simulink model "Controllo_Dinamica_Inversa_Spazio_Operativo"  (R2023a)
settings: Solver=VariableStepAuto  StartTime=0.0  StopTime=113  RelTol=1e-3
values from neighbouring files (symbols this model uses):
  a1 = 0.5    [Progetto_FoR.m]
  d0 = 1    [Progetto_FoR.m]
  KD4 = diag(kd4)    [Progetto_FoR.m]
  KI = diag(ki)    [Progetto_FoR.m]
  KP4 = diag(kp4)    [Progetto_FoR.m]
  pi0 = [ml1 Il1 Im1 Fm1 ml2 Il2 Im2 Fm2 ml3 Im3 Fm3 Il4 Im4 Fm4]    [Progetto_FoR.m]
  q0 = [0 pi/2 0 pi/2]    [Progetto_FoR.m]
  Tc = 0.001    [Progetto_FoR.m]
settings Model: Creator=panto  LastModifiedBy=panto

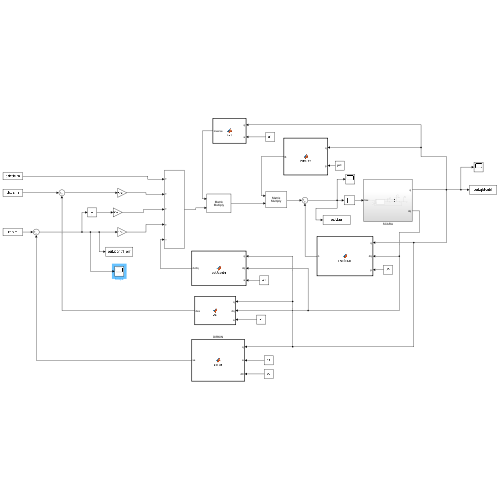
[thumbnail: Simulink's stored preview of the top-level diagram]
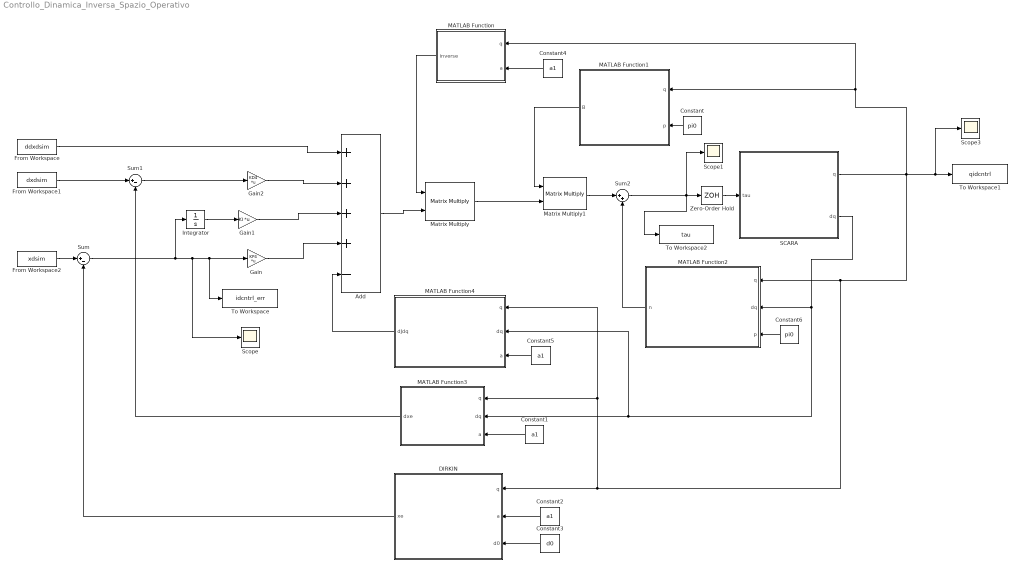
== system Controllo_Dinamica_Inversa_Spazio_Operativo ==
  Add : Sum  Inputs=++++-
  Constant : Constant  Value=pi0
  Constant{1..2,4..5} (4 alike) : Constant  Value=a1
  Constant3 : Constant  Value=d0
  Constant6 : Constant  Value=pi0
  DIRKIN : MATLAB Function  TreatAsAtomicUnit=on
  From Workspace : FromWorkspace  VariableName=ddxdsim  SampleTime=Tc
  From Workspace1 : FromWorkspace  VariableName=dxdsim  SampleTime=Tc
  From Workspace2 : FromWorkspace  VariableName=xdsim  SampleTime=Tc
  Gain : Gain  Gain=KP4  Multiplication=Matrix(K*u)
  Gain1 : Gain  Gain=KI  Multiplication=Matrix(K*u)
  Gain2 : Gain  Gain=KD4  Multiplication=Matrix(K*u)
  Integrator : Integrator
  MATLAB Function : MATLAB Function  TreatAsAtomicUnit=on
  MATLAB Function1 : MATLAB Function  TreatAsAtomicUnit=on
  MATLAB Function2 : MATLAB Function  TreatAsAtomicUnit=on
  MATLAB Function3 : MATLAB Function  TreatAsAtomicUnit=on
  MATLAB Function4 : MATLAB Function  TreatAsAtomicUnit=on
  Matrix Multiply : Product  Multiplication=Matrix(*)
  Matrix Multiply1 : Product  Multiplication=Matrix(*)
  SCARA : Subsystem
  Scope : Scope
  Scope1 : Scope
  Scope3 : Scope
  Sum : Sum  Inputs=|+-
  Sum1 : Sum  Inputs=|+-
  Sum2 : Sum  Inputs=|++
  To Workspace : ToWorkspace  VariableName=idcntrl_err  SampleTime=-1
      settings: Save2DSignal=2-D array (concatenate along first dimension)
  To Workspace1 : ToWorkspace  VariableName=qidcntrl  SampleTime=-1
      settings: Save2DSignal=2-D array (concatenate along first dimension)
  To Workspace2 : ToWorkspace  VariableName=tau  SampleTime=Tc
      settings: Save2DSignal=2-D array (concatenate along first dimension)
  Zero-Order Hold : ZeroOrderHold  SampleTime=Tc
  wires:
  Constant4/1 -> MATLAB Function/2(a)
  Constant2/1 -> DIRKIN/2(a)
  SCARA/1(q) -> MATLAB Function/1(q), MATLAB Function1/1(q), Scope3/1, To Workspace1/1, MATLAB Function3/1(q), MATLAB Function4/1(q), DIRKIN/1(q), MATLAB Function2/1(q)
  Constant3/1 -> DIRKIN/3(d0)
  DIRKIN/1(xe) -> Sum/2
  From Workspace1/1 -> Sum1/1
  Sum1/1 -> Gain2/1
  Gain2/1 -> Add/2
  MATLAB Function/1(inverse) -> Matrix Multiply/1
  Add/1 -> Matrix Multiply/2
  MATLAB Function1/1(B) -> Matrix Multiply1/1
  Matrix Multiply/1 -> Matrix Multiply1/2
  Matrix Multiply1/1 -> Sum2/1
  MATLAB Function2/1(n) -> Sum2/2
  Sum2/1 -> Scope1/1, To Workspace2/1, Zero-Order Hold/1
  SCARA/2(dq) -> MATLAB Function4/2(dq), MATLAB Function3/2(dq), MATLAB Function2/2(dq)
  Constant5/1 -> MATLAB Function4/3(a)
  Constant1/1 -> MATLAB Function3/3(a)
  MATLAB Function3/1(dxe) -> Sum1/2
  From Workspace/1 -> Add/1
  From Workspace2/1 -> Sum/1
  Zero-Order Hold/1 -> SCARA/1(tau)
  Constant/1 -> MATLAB Function1/2(p)
  Constant6/1 -> MATLAB Function2/3(p)
  Sum/1 -> Integrator/1, Scope/1, To Workspace/1, Gain/1
  Gain/1 -> Add/4
  Gain1/1 -> Add/3
  MATLAB Function4/1(dJdq) -> Add/5
  Integrator/1 -> Gain1/1

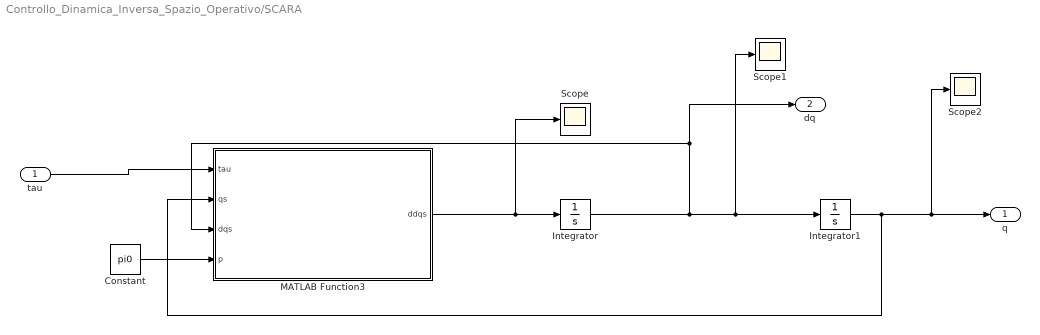
== system Controllo_Dinamica_Inversa_Spazio_Operativo/SCARA ==
  tau : Inport
  Constant : Constant  Value=pi0
  Integrator : Integrator  InitialCondition=[0;0;0;0]
  Integrator1 : Integrator  InitialCondition=q0'
  MATLAB Function3 : MATLAB Function  TreatAsAtomicUnit=on
  Scope : Scope
  Scope1 : Scope
  Scope2 : Scope
  q : Outport  SampleTime=Tc
  dq : Outport  Port=2  SampleTime=Tc
  wires:
  Integrator/1 -> dq/1, MATLAB Function3/3(dqs), Integrator1/1, Scope1/1
  tau/1 -> MATLAB Function3/1(tau)
  Integrator1/1 -> MATLAB Function3/2(qs), Scope2/1, q/1
  MATLAB Function3/1(ddqs) -> Integrator/1, Scope/1
  Constant/1 -> MATLAB Function3/4(p)

== matlab function Controllo_Dinamica_Inversa_Spazio_Operativo/DIRKIN ==
  data: q input; xe output; a input; d0 input
function xe = dirkyn(q, a, d0)
  xe = zeros(4,1);
    xe = [a*cos(q(1)+q(2))+a*cos(q(1));
        a*sin(q(1)+q(2))+a*sin(q(1));
        d0-q(3);
        q(1)+q(2)-q(4)];
end

== matlab function Controllo_Dinamica_Inversa_Spazio_Operativo/MATLAB Function ==
  data: q input; inverse output; a input
function inverse = invJ(q,a)
%devo prima calcolare lo Jacobiano analitico e poi invertirlo
%Nel caso dello SCARA, lo Jacobiano analitico coincide con quello
%geometrico: questo perchè nello SCARA l'orientamento può essere
%rappresentato direttamente dall'angolo attorno a z, e quindi la velocità
%angolare z si traduce direttamente nella velocità di cambiamento
%dell'angolo di orientamento attorno z
%dal libro when the DOFs cause rotations of the end-effector all about the 
% same fixed axis in space, the two Jacobians are essentially the same
   
    Ja = zeros(4,4);
    Ja = [-a*sin(q(1)+q(2))-a*sin(q(1)) -a*sin(q(1)+q(2)) 0 0;
        a*cos(q(1)+q(2))+a*cos(q(1)) a*cos(q(1)+q(2)) 0 0;
        0 0 -1 0;
        1 1 0 -1];

    inverse = inv(Ja);

end

== matlab function Controllo_Dinamica_Inversa_Spazio_Operativo/MATLAB Function3 ==
  data: q input; dq input; dxe output; a input
function dxe = Ja(q,dq,a)

Ja = zeros(4,4);
Ja = [-a*sin(q(1)+q(2))-a*sin(q(1)) -a*sin(q(1)+q(2)) 0 0;
        a*cos(q(1)+q(2))+a*cos(q(1)) a*cos(q(1)+q(2)) 0 0;
        0 0 -1 0;
        1 1 0 -1];

    dxe = Ja*dq;

end

== matlab function Controllo_Dinamica_Inversa_Spazio_Operativo/MATLAB Function4 ==
  data: q input; dq input; dJdq output; a input
function dJdq =  dotJadotq(q,dq,a)
    
    dotJa = zeros(4,4);
    dotJa = [-a*cos(q(1))*dq(1)-a*cos(q(1)+q(2))*(dq(1)+dq(2)) -a*cos(q(1)+q(2))*(dq(1)+dq(2)) 0 0;
        -a*sin(q(1))*dq(1)-a*sin(q(1)+q(2))*(dq(1)+dq(2)) -a*sin(q(1)+q(2))*(dq(1)+dq(2)) 0 0;
        0 0 0 0;
        0 0 0 0];

    dJdq = dotJa*dq;

end

== matlab function Controllo_Dinamica_Inversa_Spazio_Operativo/MATLAB Function1 ==
  data: q input; B output; p input
function B = Bmatrix(q,p)
%funzioni per il calcolo della matrice di inerzia
%I valori numerici sono i valori delle costanti del modello
   %funzioni per il calcolo della matrice di inerzia
%I valori numerici sono i valori delle costanti del modello
    mp = 0; %Payload
     b11 = p(2)+p(6)+p(12)+p(1)*0.0625+p(5)*(0.25+0.0625+0.25*cos(q(2))) + p(9)*(0.5+0.5*cos(q(2)))+p(3);
    b22 = p(6) + p(12) + p(5)*0.0625 + p(9)*0.25 + p(7);
    b33 = p(9) +2500*p(10);
    b44 = p(12) + 400*p(13);
    b12 = p(2) + p(12) + p(5)*(0.0625+0.125*cos(q(2))) + p(9)*(0.25+0.25*cos(q(2)));
    b21 = b12;
    b14 = -p(12);
    b41 = b14;
    b24 = b14;
    b42 = b14;

    B = [b11 b12 0 b14;
        b21 b22 0 b24;
        0 0 b33 0;
        b41 b42 0 b44];

end

== matlab function Controllo_Dinamica_Inversa_Spazio_Operativo/MATLAB Function2 ==
  data: q input; n output; dq input; p input
function n = nonlinear(q,dq,p)

mp = 0;  %massa di un eventuale carico in punta
k = -p(5)*0.125*sin(q(2)) - (p(9)+mp)*0.25*sin(q(2)); %costante per la matrice C
gr = 9.81;
g = [0; 0; -gr*(p(9)+mp); 0];

%Matrice degli attriti viscosi
f_v = [p(4) p(8) 2500*p(11) 400*p(14)];
F_v = diag(f_v);

C = [k*dq(2) k*(dq(1)+dq(2)) 0 0;
    -k*dq(1) 0 0 0;
    0 0 0 0;
    0 0 0 0];

n = C*dq +F_v*dq +g;

end

== matlab function Controllo_Dinamica_Inversa_Spazio_Operativo/SCARA/MATLAB Function3 ==
  data: tau input; ddqs output; qs input; dqs input; p input
function ddqs = SCARA(tau,qs,dqs,p)
     %devo implementare l'equazione ddq = B^-1 (tau-tau')
    %inizio calcolando B
    b11 = p(2)+p(6)+p(12)+p(1)*0.0625+p(5)*(0.25+0.0625+0.25*cos(qs(2))) + p(9)*(0.5+0.5*cos(qs(2)))+p(3);
    b22 = p(6) + p(12) + p(5)*0.0625 + p(9)*0.25 + p(7);
    b33 = p(9) +2500*p(10);
    b44 = p(12) + 400*p(13);
    b12 = p(2) + p(12) + p(5)*(0.0625+0.125*cos(qs(2))) + p(9)*(0.25+0.25*cos(qs(2)));
    b21 = b12;
    b14 = -p(12);
    b41 = b14;
    b24 = b14;
    b42 = b14;
    
    B = [b11 b12 0 b14;
        b21 b22 0 b24;
        0 0 b33 0;
        b41 b42 0 b44];
    %poi mi servono C, Fv e gravità

    k = -p(5)*0.125*sin(qs(2)) - p(9)*0.25*sin(qs(2)); %costante per la matrice C
    gr = 9.81;
    mp = 3; %Payload
    g = [0; 0; -gr*(p(9)+mp); 0];

    %Matrice degli attriti viscosi
    f_v = [0.00005 0.00005 25 2];
    F_v = diag(f_v);

    C = [k*dqs(2) k*(dqs(1)+dqs(2)) 0 0;
         -k*dqs(1) 0 0 0;
            0 0 0 0;
            0 0 0 0];
    
    tau_primo = C*dqs+F_v*dqs +g;
   
    ddqs = inv(B)*(tau-tau_primo);


end
